simulink model "PIDControllerDesign"  (R2022b)
settings: Solver=FixedStepAuto  StartTime=0.0  StopTime=10.0  FixedStep=0.01  RelTol=1e-3
values from neighbouring files (symbols this model uses):
  K = 0.6252    [ControllerDesign.m]    (also in ControllerKandT.m = 2.12; KandT.m = 1:1:length(DYawRate); PoleCancelation.m = abs(1/((scl)*(0.15*scl+1))/(2.12*(scl+a))))
  T = 0.4    [ControllerDesign.m]    (also in ControllerKandT.m = 0.15; KandT.m = 1:1:length(Dyaw_accel); csvConversion.m = 0.025; parameterCalculations.m)
settings Model: Creator=ruben  LastModifiedBy=ruben

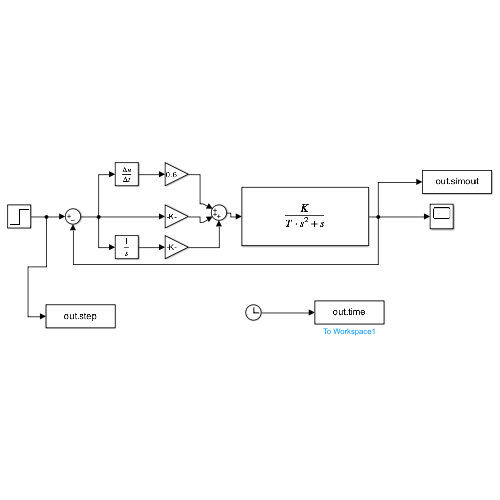
[thumbnail: Simulink's stored preview of the top-level diagram]
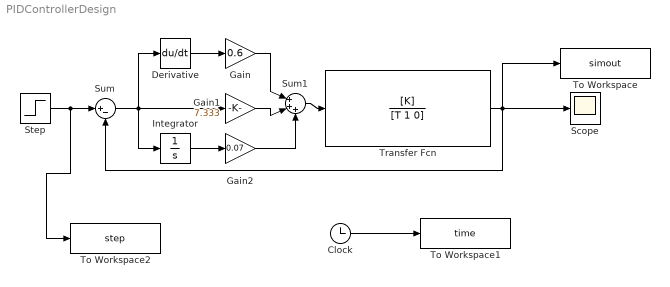
== system PIDControllerDesign ==
  Clock : Clock
  Derivative : Derivative
  Gain : Gain  Gain=0.6
  Gain1 : Gain  Gain=7.333
  Gain2 : Gain  Gain=0.07
  Integrator : Integrator
  Scope : Scope
  Step : Step  SampleTime=0
  Sum : Sum  Inputs=|+-
  Sum1 : Sum  Inputs=|+++
  To Workspace : ToWorkspace  VariableName=simout  SaveFormat=Timeseries  SampleTime=-1
  To Workspace1 : ToWorkspace  VariableName=time  SaveFormat=Timeseries  SampleTime=-1
  To Workspace2 : ToWorkspace  VariableName=step  SaveFormat=Timeseries  SampleTime=-1
  Transfer Fcn : TransferFcn  Numerator=[K]  Denominator=[T 1 0]
  wires:
  Transfer Fcn/1 -> Sum/2, To Workspace/1, Scope/1
  Step/1 -> To Workspace2/1, Sum/1
  Sum1/1 -> Transfer Fcn/1
  Sum/1 -> Derivative/1, Gain1/1, Integrator/1
  Integrator/1 -> Gain2/1
  Gain2/1 -> Sum1/3
  Gain1/1 -> Sum1/2
  Gain/1 -> Sum1/1
  Derivative/1 -> Gain/1
  Clock/1 -> To Workspace1/1
